simulink model "simu_ma"  (R2021a)
settings: Solver=VariableStepAuto  StartTime=0.0  StopTime=48387  RelTol=1e-3
settings Model: Creator=jricl  LastModifiedBy=jricl

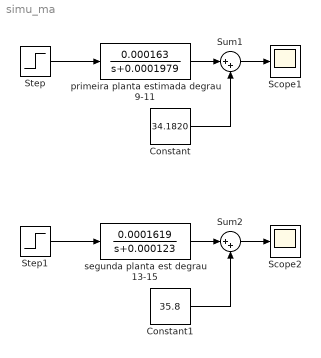
== system simu_ma ==
  Constant : Constant  Value=34.1820
  Constant1 : Constant  Value=35.8
  Scope1 : Scope
  Scope2 : Scope
  Step : Step  Time=0  After=2  SampleTime=1
  Step1 : Step  Time=0  After=2  SampleTime=1
  Sum1 : Sum  Inputs=|++
  Sum2 : Sum  Inputs=|++
  primeira planta estimada degrau 9-11 : TransferFcn  Numerator=[0.000163]  Denominator=[1 0.0001979]
  segunda planta est degrau 13-15 : TransferFcn  Numerator=[0.0001619]  Denominator=[1 0.000123]
  wires:
  primeira planta estimada degrau 9-11/1 -> Sum1/1
  Sum1/1 -> Scope1/1
  Constant/1 -> Sum1/2
  Step/1 -> primeira planta estimada degrau 9-11/1
  Step1/1 -> segunda planta est degrau 13-15/1
  Constant1/1 -> Sum2/2
  Sum2/1 -> Scope2/1
  segunda planta est degrau 13-15/1 -> Sum2/1
